simulink model "PolePlacementNonlinear"  (R2012b)
settings: Solver=ode5  StartTime=0.0  StopTime=STOP  FixedStep=T  RelTol=1e-3
values from neighbouring files (symbols this model uses):
  B = 0.1    [PolePlacement_m.m]
  comp2Den = conv([1 0],[1 100])    [PolePlacement_m.m]
  comp2Num = conv([1 10+1i*10],[1 10-1i*10])    [PolePlacement_m.m]
  dDen = dDen{1}    [PolePlacement_m.m]
  dNum = dNum{1}    [PolePlacement_m.m]
  g = 9.8    [PolePlacement_m.m]
  I = 0.006    [PolePlacement_m.m]
  K = 500    [PolePlacement_m.m]
  l = 0.3    [PolePlacement_m.m]
  m = 0.2    [PolePlacement_m.m]
  M = 0.5    [PolePlacement_m.m]
  T = .01    (= 0.01)    [PolePlacement_m.m]
  thetaInit = .2    (= 0.2)    [PolePlacement_m.m]
settings Model: Creator=Andrew  LastModifiedBy=Andrew

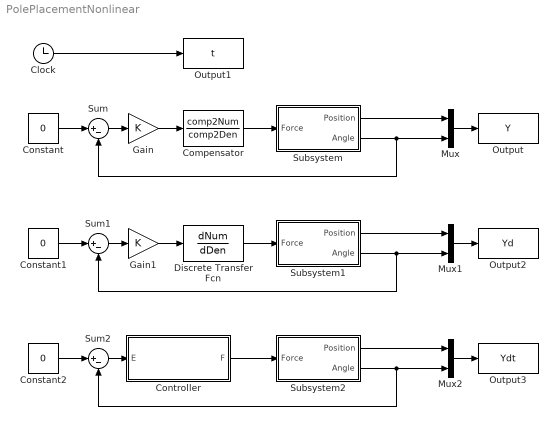
== system PolePlacementNonlinear ==
  Clock : Clock
  Compensator : TransferFcn  Numerator=comp2Num  Denominator=comp2Den
  Constant : Constant  Value=0
  Constant1 : Constant  Value=0
  Constant2 : Constant  Value=0
  Controller : Subsystem
  Discrete Transfer Fcn : DiscreteTransferFcn  Numerator=dNum  Denominator=dDen  SampleTime=T
  Gain : Gain  Gain=K
  Gain1 : Gain  Gain=K
  Mux : Mux  Inputs=2
  Mux1 : Mux  Inputs=2
  Mux2 : Mux  Inputs=2
  Output : ToWorkspace  VariableName=Y  SampleTime=-1
  Output1 : ToWorkspace  VariableName=t  SampleTime=-1
  Output2 : ToWorkspace  VariableName=Yd  SampleTime=-1
  Output3 : ToWorkspace  VariableName=Ydt  SampleTime=-1
  Subsystem : Subsystem
  Subsystem1 : Subsystem
  Subsystem2 : Subsystem
  Sum : Sum  Inputs=|+-
  Sum1 : Sum  Inputs=|+-
  Sum2 : Sum  Inputs=|+-
  wires:
  Constant/1 -> Sum/1
  Clock/1 -> Output1/1
  Mux/1 -> Output/1
  Compensator/1 -> Subsystem/1(Force)
  Subsystem/1(Position) -> Mux/1
  Subsystem/2(Angle) -> Sum/2, Mux/2
  Sum/1 -> Gain/1
  Gain/1 -> Compensator/1
  Constant1/1 -> Sum1/1
  Mux1/1 -> Output2/1
  Discrete Transfer Fcn/1 -> Subsystem1/1(Force)
  Subsystem1/1(Position) -> Mux1/1
  Subsystem1/2(Angle) -> Sum1/2, Mux1/2
  Sum1/1 -> Gain1/1
  Gain1/1 -> Discrete Transfer Fcn/1
  Constant2/1 -> Sum2/1
  Mux2/1 -> Output3/1
  Controller/1(F) -> Subsystem2/1(Force)
  Subsystem2/1(Position) -> Mux2/1
  Subsystem2/2(Angle) -> Sum2/2, Mux2/2
  Sum2/1 -> Controller/1(E)

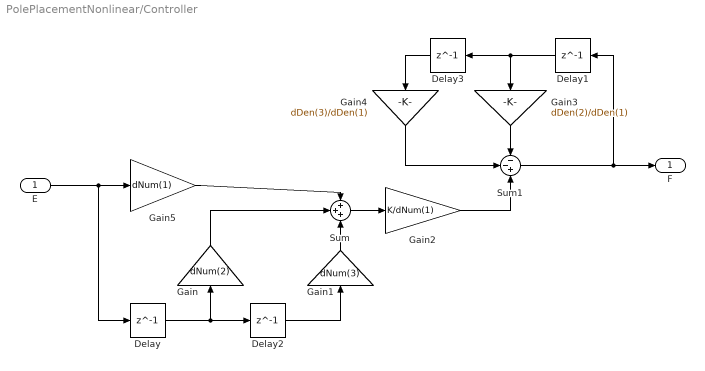
== system PolePlacementNonlinear/Controller ==
  E : Inport
  Delay{,1..3} (4 alike) : Delay  DelayLength=1  InitialCondition=0
  Gain : Gain  Gain=dNum(2)
  Gain1 : Gain  Gain=dNum(3)
  Gain2 : Gain  Gain=K/dNum(1)
  Gain3 : Gain  Gain=dDen(2)/dDen(1)
  Gain4 : Gain  Gain=dDen(3)/dDen(1)
  Gain5 : Gain  Gain=dNum(1)
  Sum : Sum  Inputs=+++
  Sum1 : Sum  Inputs=--+
  F : Outport
  wires:
  E/1 -> Gain5/1, Delay/1
  Delay/1 -> Delay2/1, Gain/1
  Delay2/1 -> Gain1/1
  Gain/1 -> Sum/2
  Gain1/1 -> Sum/3
  Sum/1 -> Gain2/1
  Gain2/1 -> Sum1/3
  Sum1/1 -> F/1, Delay1/1
  Delay3/1 -> Gain4/1
  Delay1/1 -> Delay3/1, Gain3/1
  Gain3/1 -> Sum1/1
  Gain4/1 -> Sum1/2
  Gain5/1 -> Sum/1

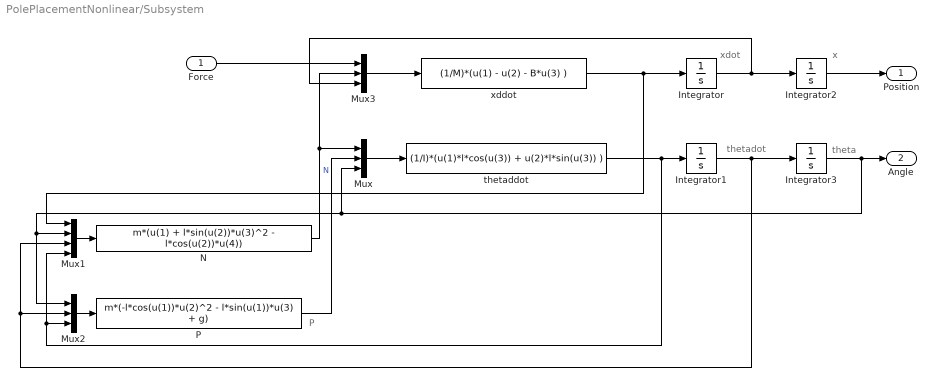
== system PolePlacementNonlinear/Subsystem ==
  note: xdot
  note: x
  note: thetadot
  note: theta
  note: P
  Force : Inport
  Integrator : Integrator  ContinuousStateAttributes='xdot'
  Integrator1 : Integrator  ContinuousStateAttributes='thetadot'
  Integrator2 : Integrator  ContinuousStateAttributes='x'
  Integrator3 : Integrator  InitialCondition=thetaInit  ContinuousStateAttributes='theta'
  Mux : Mux  Inputs=3
  Mux1 : Mux
  Mux2 : Mux  Inputs=3
  Mux3 : Mux  Inputs=3
  N : Fcn  Expr=m*(u(1) + l*sin(u(2))*u(3)^2 - l*cos(u(2))*u(4))
  P : Fcn  Expr=m*(-l*cos(u(1))*u(2)^2 - l*sin(u(1))*u(3) + g)
  thetaddot : Fcn  Expr=(1/I)*(u(1)*l*cos(u(3)) + u(2)*l*sin(u(3)) )
  xddot : Fcn  Expr=(1/M)*(u(1) - u(2) - B*u(3) )
  Position : Outport
  Angle : Outport  Port=2
  wires:
  Integrator/1 -> Integrator2/1, Mux3/3
  Integrator1/1 -> Mux1/3, Mux2/2, Integrator3/1
  xddot/1 -> Integrator/1, Mux1/1
  thetaddot/1 -> Mux1/4, Mux2/3, Integrator1/1
  Mux/1 -> thetaddot/1
  Integrator2/1 -> Position/1
  Integrator3/1 -> Mux2/1, Mux1/2, Mux/3, Angle/1
  Mux1/1 -> N/1
  Mux3/1 -> xddot/1
  Force/1 -> Mux3/1
  N/1 -> Mux/1, Mux3/2  "N"
  Mux2/1 -> P/1
  P/1 -> Mux/2

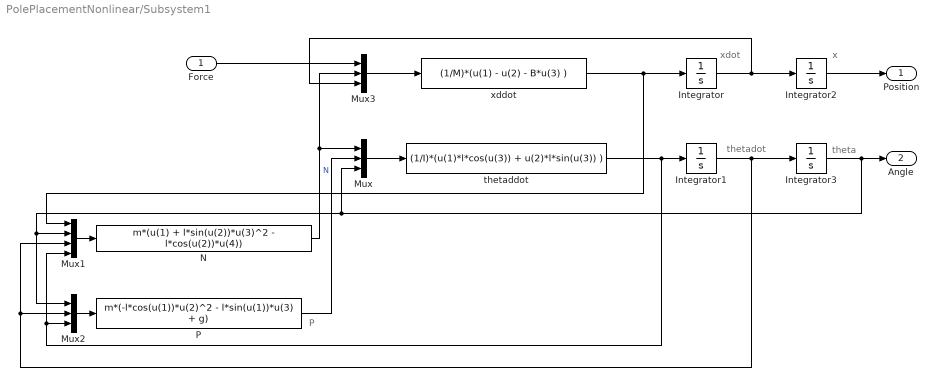
== system PolePlacementNonlinear/Subsystem1 ==
  note: xdot
  note: x
  note: thetadot
  note: theta
  note: P
  Force : Inport
  Integrator : Integrator  ContinuousStateAttributes='xdot'
  Integrator1 : Integrator  ContinuousStateAttributes='thetadot'
  Integrator2 : Integrator  ContinuousStateAttributes='x'
  Integrator3 : Integrator  InitialCondition=thetaInit  ContinuousStateAttributes='theta'
  Mux : Mux  Inputs=3
  Mux1 : Mux
  Mux2 : Mux  Inputs=3
  Mux3 : Mux  Inputs=3
  N : Fcn  Expr=m*(u(1) + l*sin(u(2))*u(3)^2 - l*cos(u(2))*u(4))
  P : Fcn  Expr=m*(-l*cos(u(1))*u(2)^2 - l*sin(u(1))*u(3) + g)
  thetaddot : Fcn  Expr=(1/I)*(u(1)*l*cos(u(3)) + u(2)*l*sin(u(3)) )
  xddot : Fcn  Expr=(1/M)*(u(1) - u(2) - B*u(3) )
  Position : Outport
  Angle : Outport  Port=2
  wires:
  Integrator/1 -> Integrator2/1, Mux3/3
  Integrator1/1 -> Mux1/3, Mux2/2, Integrator3/1
  xddot/1 -> Integrator/1, Mux1/1
  thetaddot/1 -> Mux1/4, Mux2/3, Integrator1/1
  Mux/1 -> thetaddot/1
  Integrator2/1 -> Position/1
  Integrator3/1 -> Mux2/1, Mux1/2, Mux/3, Angle/1
  Mux1/1 -> N/1
  Mux3/1 -> xddot/1
  Force/1 -> Mux3/1
  N/1 -> Mux/1, Mux3/2  "N"
  Mux2/1 -> P/1
  P/1 -> Mux/2

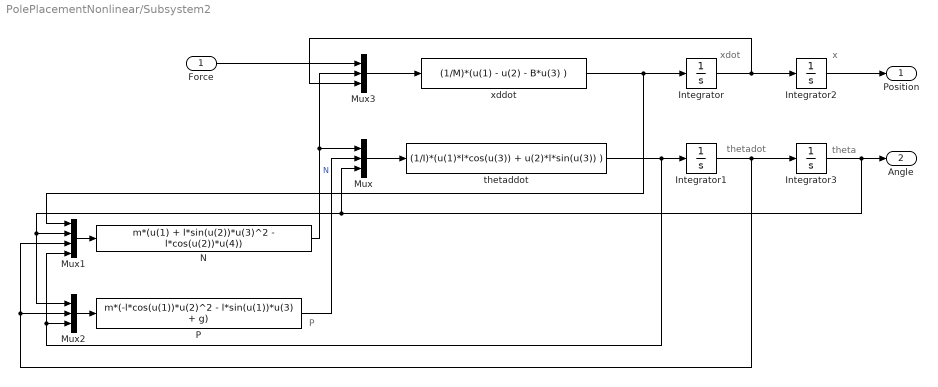
== system PolePlacementNonlinear/Subsystem2 ==
  note: xdot
  note: x
  note: thetadot
  note: theta
  note: P
  Force : Inport
  Integrator : Integrator  ContinuousStateAttributes='xdot'
  Integrator1 : Integrator  ContinuousStateAttributes='thetadot'
  Integrator2 : Integrator  ContinuousStateAttributes='x'
  Integrator3 : Integrator  InitialCondition=thetaInit  ContinuousStateAttributes='theta'
  Mux : Mux  Inputs=3
  Mux1 : Mux
  Mux2 : Mux  Inputs=3
  Mux3 : Mux  Inputs=3
  N : Fcn  Expr=m*(u(1) + l*sin(u(2))*u(3)^2 - l*cos(u(2))*u(4))
  P : Fcn  Expr=m*(-l*cos(u(1))*u(2)^2 - l*sin(u(1))*u(3) + g)
  thetaddot : Fcn  Expr=(1/I)*(u(1)*l*cos(u(3)) + u(2)*l*sin(u(3)) )
  xddot : Fcn  Expr=(1/M)*(u(1) - u(2) - B*u(3) )
  Position : Outport
  Angle : Outport  Port=2
  wires:
  Integrator/1 -> Integrator2/1, Mux3/3
  Integrator1/1 -> Mux1/3, Mux2/2, Integrator3/1
  xddot/1 -> Integrator/1, Mux1/1
  thetaddot/1 -> Mux1/4, Mux2/3, Integrator1/1
  Mux/1 -> thetaddot/1
  Integrator2/1 -> Position/1
  Integrator3/1 -> Mux2/1, Mux1/2, Mux/3, Angle/1
  Mux1/1 -> N/1
  Mux3/1 -> xddot/1
  Force/1 -> Mux3/1
  N/1 -> Mux/1, Mux3/2  "N"
  Mux2/1 -> P/1
  P/1 -> Mux/2
